simulink model "gg_plus_lc_platoon"  (R2019a)
settings: Solver=ode23t  StartTime=0.0  StopTime=70  FixedStep=0.1  MaxStep=0.01  RelTol=1e-3
InitFcn:
  | load vehStatesBus
libraries: simulink x120, powerlib_meascontrol x14, dspsigops x7, autolibshared x7
(part 1 of 7)
settings Model: Creator=fvall  LastModifiedBy=fvall
settings DebuggingCC: ReadBeforeWriteMsg=DisableAll  WriteAfterWriteMsg=DisableAll  WriteAfterReadMsg=DisableAll  MultiTaskDSMMsg=none
settings ModelReferenceCC: UpdateModelReferenceTargets=IfOutOfDate
settings SFSimCC: SFSimEcho=off

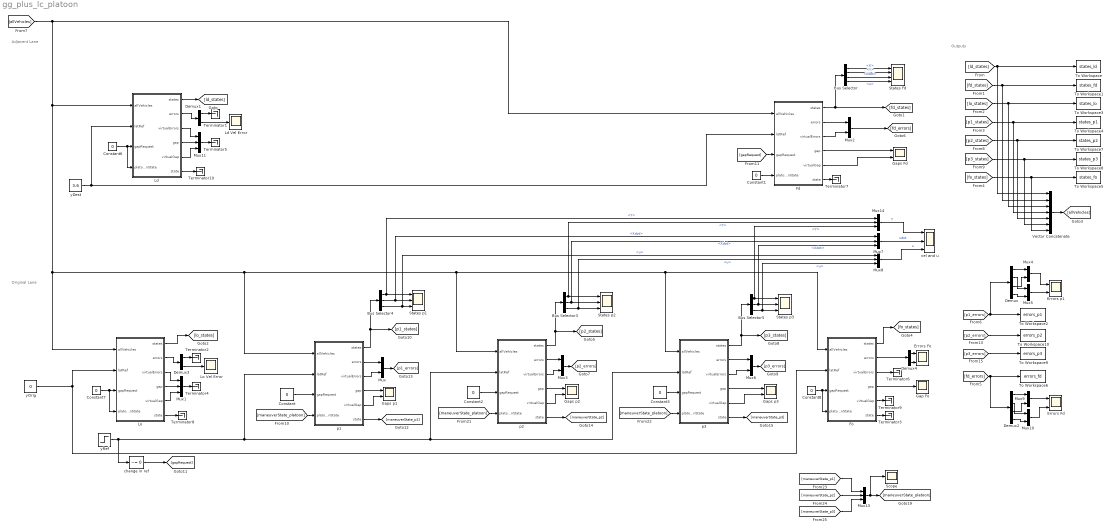
== system gg_plus_lc_platoon ==
  note: Adjacent Lane
  note: Outputs
  note: Original Lane
  Bus Selector : BusSelector  OutputSignals=X,Y,Xdot,u
  Bus Selector3 : BusSelector  OutputSignals=Y,Xdot,u
  Bus Selector4 : BusSelector  OutputSignals=Y,Xdot,u
  Bus Selector5 : BusSelector  OutputSignals=Y,Xdot,u
  Constant{,1..3,6..8} (7 alike) : Constant  Value=0
  Demux : Demux
  Demux1 : Demux  Outputs=2
  Demux2 : Demux
  Demux3 : Demux  Outputs=2
  Demux4 : Demux  Outputs=2
  Errors Fd : Scope  NumInputPorts=2
  Errors Fo : Scope  NumInputPorts=2
  Errors p1 : Scope  NumInputPorts=2
  Fd : Subsystem  mask{m=2000, lf=2.5, lr=2.5, maxAcceleration=4, minAcceleration=-8, maxJerk=40, minJerk=-50, maxDelta=0.43633, maxDeltaDot=0.16406, freeFlowVel=25, posInPlatoon=1, A=[0 1 25 0;0 -0.92 0 -25.1;0 0 0 1;0 -0.05 0 -2.875], B=[0;12;0;15], C=[1 0 0 0;0 0 0 1], x0=62.7512, vx0=25, y0=3.6, h=0.63, d0=0.5004, minHeadwayError=-100, maxHeadwayError=3, velFilterGain=10, Kd=1.5652, Kp=2.2775, Ki=0.75, velKi=0.5, velKp=1.5, hFilterGain=1, hFilterSaturation=0.5, vMin=16.25, maxComfAccel=2, minComfAccel=-2, maxComfJerk=10, minComfJerk=-10, strategy=2, hLc=1.9025, d0Lc=0.5004, Klat=[0.00909090909090922 0.00739381562390402 0.848484848484842 0.174418280834209], L=[12.1618468638973 6.0911647386398;-3.34743889176456 -72.8238882817198;1.29674659792577 4.97919690407453;0.0997536738638272 3.54315313610273]}
      mask prompts: m "autoblks_shared:autoblkVehBody3DofLat:blkPrm_m"; lf "autoblks_shared:autoblkVehBody3DofLat:blkPrm_a"; lr "autoblks_shared:autoblkVehBody3DofLat:blkPrm_b"; maxAcceleration "Max Acceleration"; minAcceleration "Min Acceleration"; maxJerk "Max Jerk"; minJerk "Min Jerk"; maxDelta "Max Delta"; maxDeltaDot "Max Delta Dot"; freeFlowVel "Free Flow Velocity"; posInPlatoon "Position in Platoon"; x0 "autoblks_shared:autoblkVehBody3DofLat:blkPrm_X_o"; vx0 "autoblks_shared:autoblkVehBody3DofLat:blkPrm_xdot_o"; y0 "autoblks_shared:autoblkVehBody3DofLat:blkPrm_Y_o"; h "Time Headway"; d0 "Standstill Gap"; minHeadwayError "Min Headway Error"; maxHeadwayError "Max Headway Error"; velFilterGain "Velocity Filter Gain"; hFilterGain "Headway Filter Gain"; hFilterSaturation "Headway Filter Saturation"; vMin "Min Velocity"; maxComfAccel "Max Comf Accel"; minComfAccel "Min Comf Accel"; maxComfJerk "Max Comf Jerk"; minComfJerk "Min Comf Jerk"; strategy "LC strategy"; hLc "Time Headway LC"; d0Lc "Standstill Gap LC"; Klat "Lat Controller Gain"; L "Observer Gain"
      mask TypeOptions m: Vehicle Body 3DOF Single Track/m
      mask TypeOptions lf: Vehicle Body 3DOF Single Track/a
      mask TypeOptions lr: Vehicle Body 3DOF Single Track/b
      mask TypeOptions maxDelta: Lateral Control/Saturation/UpperLimit
      mask TypeOptions maxDeltaDot: Lateral Control/Rate Limiter/RisingSlewLimit
      mask TypeOptions posInPlatoon: posInPlatoon/Value
      mask TypeOptions A:
      | Lateral Control/Full State
      | Observer/Gain3/Gain
      mask TypeOptions B:
      | Lateral Control/Full State
      | Observer/Gain/Gain
      mask TypeOptions C:
      | Lateral Control/Full State
      | Observer/Gain1/Gain
      mask TypeOptions x0: Vehicle Body 3DOF Single Track/X_o
      mask TypeOptions vx0: Vehicle Body 3DOF Single Track/xdot_o
      mask TypeOptions y0: Vehicle Body 3DOF Single Track/Y_o
      mask TypeOptions h:
      | Regular Vehicle
      | Following/Compute Errors/h/Value
      mask TypeOptions d0:
      | Regular Vehicle
      | Following/Compute Errors/d0/Value
      mask TypeOptions strategy: strategy/Value
      mask TypeOptions Klat: Lateral Control/Gain1/Gain
      mask TypeOptions L:
      | Lateral Control/Full State
      | Observer/Gain2/Gain
      mask DialogControl DescGroupVar Prompt: 3DOF Vehicle with ACC
      mask DialogControl DescTextVar Prompt: Vehicle with ACC. The vehicle model is Simulink's 3DOF single track vehicle body. The controller is a PID with constant headway including headway error saturation and filtered leader velocity.
      mask DialogControl VehParams Prompt: Vehicle Parameters
      mask DialogControl m Prompt: Vehicle mass, m [kg]:
      mask DialogControl lf Prompt: Longitudinal distance from center of mass to front axle, a [m]:
      mask DialogControl lr Prompt: Longitudinal distance from center of mass to rear axle, b [m]:
      mask DialogControl latLinearModel Prompt: Lat Linear Model
      mask DialogControl InitStates Prompt: Initial State
      mask DialogControl x0 Prompt: Initial inertial frame longitudinal position, X_o [m]:
      mask DialogControl vx0 Prompt: Initial longitudinal velocity, xdot_o [m/s]:
      mask DialogControl y0 Prompt: Initial inertial frame lateral displacement, Y_o [m]:
      mask DialogControl Container3 Prompt: Veh Following Parameters
      mask DialogControl VirtualFollParams Prompt: Virtual Veh Following Parameters
      mask DialogControl LCParams Prompt: Lane Change Params
  Fo : Subsystem  mask{m=2000, lf=2.5, lr=2.5, maxAcceleration=4, minAcceleration=-8, maxJerk=40, minJerk=-50, maxDelta=0.43633, maxDeltaDot=0.16406, freeFlowVel=25, posInPlatoon=1, A=[0 1 25 0;0 -0.92 0 -25.1;0 0 0 1;0 -0.05 0 -2.875], B=[0;12;0;15], C=[1 0 0 0;0 0 0 1], x0=0, vx0=25, y0=0, h=0.63, d0=0.5004, minHeadwayError=-100, maxHeadwayError=3, velFilterGain=10, Kd=1.5652, Kp=2.2775, Ki=0.75, velKi=0.5, velKp=1.5, hFilterGain=1, hFilterSaturation=0.5, vMin=16.25, maxComfAccel=2, minComfAccel=-2, maxComfJerk=10, minComfJerk=-10, strategy=2, hLc=1.9025, d0Lc=0.5004, Klat=[0.00909090909090922 0.00739381562390402 0.848484848484842 0.174418280834209], L=[12.1618468638973 6.0911647386398;-3.34743889176456 -72.8238882817198;1.29674659792577 4.97919690407453;0.0997536738638272 3.54315313610273]}
      mask prompts: m "autoblks_shared:autoblkVehBody3DofLat:blkPrm_m"; lf "autoblks_shared:autoblkVehBody3DofLat:blkPrm_a"; lr "autoblks_shared:autoblkVehBody3DofLat:blkPrm_b"; maxAcceleration "Max Acceleration"; minAcceleration "Min Acceleration"; maxJerk "Max Jerk"; minJerk "Min Jerk"; maxDelta "Max Delta"; maxDeltaDot "Max Delta Dot"; freeFlowVel "Free Flow Velocity"; posInPlatoon "Position in Platoon"; x0 "autoblks_shared:autoblkVehBody3DofLat:blkPrm_X_o"; vx0 "autoblks_shared:autoblkVehBody3DofLat:blkPrm_xdot_o"; y0 "autoblks_shared:autoblkVehBody3DofLat:blkPrm_Y_o"; h "Time Headway"; d0 "Standstill Gap"; minHeadwayError "Min Headway Error"; maxHeadwayError "Max Headway Error"; velFilterGain "Velocity Filter Gain"; hFilterGain "Headway Filter Gain"; hFilterSaturation "Headway Filter Saturation"; vMin "Min Velocity"; maxComfAccel "Max Comf Accel"; minComfAccel "Min Comf Accel"; maxComfJerk "Max Comf Jerk"; minComfJerk "Min Comf Jerk"; strategy "LC strategy"; hLc "Time Headway LC"; d0Lc "Standstill Gap LC"; Klat "Lat Controller Gain"; L "Observer Gain"
      mask TypeOptions m: Vehicle Body 3DOF Single Track/m
      mask TypeOptions lf: Vehicle Body 3DOF Single Track/a
      mask TypeOptions lr: Vehicle Body 3DOF Single Track/b
      mask TypeOptions maxDelta: Lateral Control/Saturation/UpperLimit
      mask TypeOptions maxDeltaDot: Lateral Control/Rate Limiter/RisingSlewLimit
      mask TypeOptions posInPlatoon: posInPlatoon/Value
      mask TypeOptions A:
      | Lateral Control/Full State
      | Observer/Gain3/Gain
      mask TypeOptions B:
      | Lateral Control/Full State
      | Observer/Gain/Gain
      mask TypeOptions C:
      | Lateral Control/Full State
      | Observer/Gain1/Gain
      mask TypeOptions x0: Vehicle Body 3DOF Single Track/X_o
      mask TypeOptions vx0: Vehicle Body 3DOF Single Track/xdot_o
      mask TypeOptions y0: Vehicle Body 3DOF Single Track/Y_o
      mask TypeOptions h:
      | Regular Vehicle
      | Following/Compute Errors/h/Value
      mask TypeOptions d0:
      | Regular Vehicle
      | Following/Compute Errors/d0/Value
      mask TypeOptions strategy: strategy/Value
      mask TypeOptions Klat: Lateral Control/Gain1/Gain
      mask TypeOptions L:
      | Lateral Control/Full State
      | Observer/Gain2/Gain
      mask DialogControl DescGroupVar Prompt: 3DOF Vehicle with ACC
      mask DialogControl DescTextVar Prompt: Vehicle with ACC. The vehicle model is Simulink's 3DOF single track vehicle body. The controller is a PID with constant headway including headway error saturation and filtered leader velocity.
      mask DialogControl VehParams Prompt: Vehicle Parameters
      mask DialogControl m Prompt: Vehicle mass, m [kg]:
      mask DialogControl lf Prompt: Longitudinal distance from center of mass to front axle, a [m]:
      mask DialogControl lr Prompt: Longitudinal distance from center of mass to rear axle, b [m]:
      mask DialogControl latLinearModel Prompt: Lat Linear Model
      mask DialogControl InitStates Prompt: Initial State
      mask DialogControl x0 Prompt: Initial inertial frame longitudinal position, X_o [m]:
      mask DialogControl vx0 Prompt: Initial longitudinal velocity, xdot_o [m/s]:
      mask DialogControl y0 Prompt: Initial inertial frame lateral displacement, Y_o [m]:
      mask DialogControl Container3 Prompt: Veh Following Parameters
      mask DialogControl VirtualFollParams Prompt: Virtual Veh Following Parameters
      mask DialogControl LCParams Prompt: Lane Change Params
  Gap Fo : Scope
  Gaps Fd : Scope  NumInputPorts=2
  Gaps p1 : Scope  NumInputPorts=2
  Gaps p2 : Scope  NumInputPorts=2
  Gaps p3 : Scope  NumInputPorts=2
  Ld : Subsystem  mask{m=2000, lf=2.5, lr=2.5, maxAcceleration=4, minAcceleration=-8, maxJerk=40, minJerk=-50, maxDelta=0.43633, maxDeltaDot=0.16406, freeFlowVel=25, posInPlatoon=1, A=[0 1 25 0;0 -0.92 0 -25.1;0 0 0 1;0 -0.05 0 -2.875], B=[0;12;0;15], C=[1 0 0 0;0 0 0 1], x0=84.0016, vx0=25, y0=3.6, h=0.63, d0=0.5004, minHeadwayError=-100, maxHeadwayError=3, velFilterGain=10, Kd=1.5652, Kp=2.2775, Ki=0.75, velKi=0.5, velKp=1.5, hFilterGain=1, hFilterSaturation=0.5, vMin=16.25, maxComfAccel=2, minComfAccel=-2, maxComfJerk=10, minComfJerk=-10, strategy=2, hLc=1.9025, d0Lc=0.5004, Klat=[0.00909090909090922 0.00739381562390402 0.848484848484842 0.174418280834209], L=[12.1618468638973 6.0911647386398;-3.34743889176456 -72.8238882817198;1.29674659792577 4.97919690407453;0.0997536738638272 3.54315313610273]}
      mask prompts: m "autoblks_shared:autoblkVehBody3DofLat:blkPrm_m"; lf "autoblks_shared:autoblkVehBody3DofLat:blkPrm_a"; lr "autoblks_shared:autoblkVehBody3DofLat:blkPrm_b"; maxAcceleration "Max Acceleration"; minAcceleration "Min Acceleration"; maxJerk "Max Jerk"; minJerk "Min Jerk"; maxDelta "Max Delta"; maxDeltaDot "Max Delta Dot"; freeFlowVel "Free Flow Velocity"; posInPlatoon "Position in Platoon"; x0 "autoblks_shared:autoblkVehBody3DofLat:blkPrm_X_o"; vx0 "autoblks_shared:autoblkVehBody3DofLat:blkPrm_xdot_o"; y0 "autoblks_shared:autoblkVehBody3DofLat:blkPrm_Y_o"; h "Time Headway"; d0 "Standstill Gap"; minHeadwayError "Min Headway Error"; maxHeadwayError "Max Headway Error"; velFilterGain "Velocity Filter Gain"; hFilterGain "Headway Filter Gain"; hFilterSaturation "Headway Filter Saturation"; vMin "Min Velocity"; maxComfAccel "Max Comf Accel"; minComfAccel "Min Comf Accel"; maxComfJerk "Max Comf Jerk"; minComfJerk "Min Comf Jerk"; strategy "LC strategy"; hLc "Time Headway LC"; d0Lc "Standstill Gap LC"; Klat "Lat Controller Gain"; L "Observer Gain"
      mask TypeOptions m: Vehicle Body 3DOF Single Track/m
      mask TypeOptions lf: Vehicle Body 3DOF Single Track/a
      mask TypeOptions lr: Vehicle Body 3DOF Single Track/b
      mask TypeOptions maxDelta: Lateral Control/Saturation/UpperLimit
      mask TypeOptions maxDeltaDot: Lateral Control/Rate Limiter/RisingSlewLimit
      mask TypeOptions posInPlatoon: posInPlatoon/Value
      mask TypeOptions A:
      | Lateral Control/Full State
      | Observer/Gain3/Gain
      mask TypeOptions B:
      | Lateral Control/Full State
      | Observer/Gain/Gain
      mask TypeOptions C:
      | Lateral Control/Full State
      | Observer/Gain1/Gain
      mask TypeOptions x0: Vehicle Body 3DOF Single Track/X_o
      mask TypeOptions vx0: Vehicle Body 3DOF Single Track/xdot_o
      mask TypeOptions y0: Vehicle Body 3DOF Single Track/Y_o
      mask TypeOptions h:
      | Regular Vehicle
      | Following/Compute Errors/h/Value
      mask TypeOptions d0:
      | Regular Vehicle
      | Following/Compute Errors/d0/Value
      mask TypeOptions strategy: strategy/Value
      mask TypeOptions Klat: Lateral Control/Gain1/Gain
      mask TypeOptions L:
      | Lateral Control/Full State
      | Observer/Gain2/Gain
      mask DialogControl DescGroupVar Prompt: 3DOF Vehicle with ACC
      mask DialogControl DescTextVar Prompt: Vehicle with ACC. The vehicle model is Simulink's 3DOF single track vehicle body. The controller is a PID with constant headway including headway error saturation and filtered leader velocity.
      mask DialogControl VehParams Prompt: Vehicle Parameters
      mask DialogControl m Prompt: Vehicle mass, m [kg]:
      mask DialogControl lf Prompt: Longitudinal distance from center of mass to front axle, a [m]:
      mask DialogControl lr Prompt: Longitudinal distance from center of mass to rear axle, b [m]:
      mask DialogControl latLinearModel Prompt: Lat Linear Model
      mask DialogControl InitStates Prompt: Initial State
      mask DialogControl x0 Prompt: Initial inertial frame longitudinal position, X_o [m]:
      mask DialogControl vx0 Prompt: Initial longitudinal velocity, xdot_o [m/s]:
      mask DialogControl y0 Prompt: Initial inertial frame lateral displacement, Y_o [m]:
      mask DialogControl Container3 Prompt: Veh Following Parameters
      mask DialogControl VirtualFollParams Prompt: Virtual Veh Following Parameters
      mask DialogControl LCParams Prompt: Lane Change Params
  Ld Vel Error : Scope
  Lo : Subsystem  mask{m=2000, lf=2.5, lr=2.5, maxAcceleration=4, minAcceleration=-8, maxJerk=40, minJerk=-50, maxDelta=0.43633, maxDeltaDot=0.16406, freeFlowVel=25, posInPlatoon=1, A=[0 1 25 0;0 -0.92 0 -25.1;0 0 0 1;0 -0.05 0 -2.875], B=[0;12;0;15], C=[1 0 0 0;0 0 0 1], x0=85.0016, vx0=25, y0=0, h=0.63, d0=0.5004, minHeadwayError=-100, maxHeadwayError=3, velFilterGain=10, Kd=1.5652, Kp=2.2775, Ki=0.75, velKi=0.5, velKp=1.5, hFilterGain=1, hFilterSaturation=0.5, vMin=16.25, maxComfAccel=2, minComfAccel=-2, maxComfJerk=10, minComfJerk=-10, strategy=2, hLc=1.9025, d0Lc=0.5004, Klat=[0.00909090909090922 0.00739381562390402 0.848484848484842 0.174418280834209], L=[12.1618468638973 6.0911647386398;-3.34743889176456 -72.8238882817198;1.29674659792577 4.97919690407453;0.0997536738638272 3.54315313610273]}
      mask prompts: m "autoblks_shared:autoblkVehBody3DofLat:blkPrm_m"; lf "autoblks_shared:autoblkVehBody3DofLat:blkPrm_a"; lr "autoblks_shared:autoblkVehBody3DofLat:blkPrm_b"; maxAcceleration "Max Acceleration"; minAcceleration "Min Acceleration"; maxJerk "Max Jerk"; minJerk "Min Jerk"; maxDelta "Max Delta"; maxDeltaDot "Max Delta Dot"; freeFlowVel "Free Flow Velocity"; posInPlatoon "Position in Platoon"; x0 "autoblks_shared:autoblkVehBody3DofLat:blkPrm_X_o"; vx0 "autoblks_shared:autoblkVehBody3DofLat:blkPrm_xdot_o"; y0 "autoblks_shared:autoblkVehBody3DofLat:blkPrm_Y_o"; h "Time Headway"; d0 "Standstill Gap"; minHeadwayError "Min Headway Error"; maxHeadwayError "Max Headway Error"; velFilterGain "Velocity Filter Gain"; hFilterGain "Headway Filter Gain"; hFilterSaturation "Headway Filter Saturation"; vMin "Min Velocity"; maxComfAccel "Max Comf Accel"; minComfAccel "Min Comf Accel"; maxComfJerk "Max Comf Jerk"; minComfJerk "Min Comf Jerk"; strategy "LC strategy"; hLc "Time Headway LC"; d0Lc "Standstill Gap LC"; Klat "Lat Controller Gain"; L "Observer Gain"
      mask TypeOptions m: Vehicle Body 3DOF Single Track/m
      mask TypeOptions lf: Vehicle Body 3DOF Single Track/a
      mask TypeOptions lr: Vehicle Body 3DOF Single Track/b
      mask TypeOptions maxDelta: Lateral Control/Saturation/UpperLimit
      mask TypeOptions maxDeltaDot: Lateral Control/Rate Limiter/RisingSlewLimit
      mask TypeOptions posInPlatoon: posInPlatoon/Value
      mask TypeOptions A:
      | Lateral Control/Full State
      | Observer/Gain3/Gain
      mask TypeOptions B:
      | Lateral Control/Full State
      | Observer/Gain/Gain
      mask TypeOptions C:
      | Lateral Control/Full State
      | Observer/Gain1/Gain
      mask TypeOptions x0: Vehicle Body 3DOF Single Track/X_o
      mask TypeOptions vx0: Vehicle Body 3DOF Single Track/xdot_o
      mask TypeOptions y0: Vehicle Body 3DOF Single Track/Y_o
      mask TypeOptions h:
      | Regular Vehicle
      | Following/Compute Errors/h/Value
      mask TypeOptions d0:
      | Regular Vehicle
      | Following/Compute Errors/d0/Value
      mask TypeOptions strategy: strategy/Value
      mask TypeOptions Klat: Lateral Control/Gain1/Gain
      mask TypeOptions L:
      | Lateral Control/Full State
      | Observer/Gain2/Gain
      mask DialogControl DescGroupVar Prompt: 3DOF Vehicle with ACC
      mask DialogControl DescTextVar Prompt: Vehicle with ACC. The vehicle model is Simulink's 3DOF single track vehicle body. The controller is a PID with constant headway including headway error saturation and filtered leader velocity.
      mask DialogControl VehParams Prompt: Vehicle Parameters
      mask DialogControl m Prompt: Vehicle mass, m [kg]:
      mask DialogControl lf Prompt: Longitudinal distance from center of mass to front axle, a [m]:
      mask DialogControl lr Prompt: Longitudinal distance from center of mass to rear axle, b [m]:
      mask DialogControl latLinearModel Prompt: Lat Linear Model
      mask DialogControl InitStates Prompt: Initial State
      mask DialogControl x0 Prompt: Initial inertial frame longitudinal position, X_o [m]:
      mask DialogControl vx0 Prompt: Initial longitudinal velocity, xdot_o [m/s]:
      mask DialogControl y0 Prompt: Initial inertial frame lateral displacement, Y_o [m]:
      mask DialogControl Container3 Prompt: Veh Following Parameters
      mask DialogControl VirtualFollParams Prompt: Virtual Veh Following Parameters
      mask DialogControl LCParams Prompt: Lane Change Params
  Lo Vel Error : Scope
  Mux{,2..6,9..10} (8 alike) : Mux  Inputs=2
  Mux{1,7..8,11,13..14} (6 alike) : Mux  Inputs=3
  Scope : Scope
  States Fd : Scope  NumInputPorts=4
  States p1 : Scope  NumInputPorts=3
  States p2 : Scope  NumInputPorts=3
  States p3 : Scope  NumInputPorts=3
  Terminator{1..10} (10 alike) : Terminator
  To Workspace : ToWorkspace  VariableName=states_ld  SaveFormat=Timeseries  SampleTime=-1
  To Workspace1 : ToWorkspace  VariableName=states_fd  SaveFormat=Timeseries  SampleTime=-1
  To Workspace10 : ToWorkspace  VariableName=errors_p2  SampleTime=-1
  To Workspace2 : ToWorkspace  VariableName=errors_p1  SampleTime=-1
  To Workspace3 : ToWorkspace  VariableName=states_lo  SaveFormat=Timeseries  SampleTime=-1
  To Workspace4 : ToWorkspace  VariableName=states_p1  SaveFormat=Timeseries  SampleTime=-1
  To Workspace5 : ToWorkspace  VariableName=states_fo  SaveFormat=Timeseries  SampleTime=-1
  To Workspace6 : ToWorkspace  VariableName=errors_fd  SampleTime=-1
  To Workspace7 : ToWorkspace  VariableName=states_p2  SaveFormat=Timeseries  SampleTime=-1
  To Workspace8 : ToWorkspace  VariableName=states_p3  SaveFormat=Timeseries  SampleTime=-1
  To Workspace9 : ToWorkspace  VariableName=errors_p3  SampleTime=-1
  Vector Concatenate : Concatenate  NumInputs=7
  change in ref : simulink/Logic and Bit Operations/Compare To Constant  relop=~=  const=0  OutDataTypeStr=boolean
  p1 : Subsystem  mask{m=2000, lf=2.5, lr=2.5, maxAcceleration=4, minAcceleration=-8, maxJerk=40, minJerk=-50, maxDelta=0.43633, maxDeltaDot=0.16406, freeFlowVel=25, posInPlatoon=1, A=[0 1 25 0;0 -0.92 0 -25.1;0 0 0 1;0 -0.05 0 -2.875], B=[0;12;0;15], C=[1 0 0 0;0 0 0 1], x0=63.7512, vx0=25, y0=0, h=0.63, d0=0.5004, minHeadwayError=-100, maxHeadwayError=3, velFilterGain=10, Kd=1.5652, Kp=2.2775, Ki=0.75, velKi=0.5, velKp=1.5, hFilterGain=1, hFilterSaturation=0.5, vMin=16.25, maxComfAccel=2, minComfAccel=-2, maxComfJerk=10, minComfJerk=-10, strategy=2, hLc=1.9025, d0Lc=0.5004, Klat=[0.00909090909090922 0.00739381562390402 0.848484848484842 0.174418280834209], L=[12.1618468638973 6.0911647386398;-3.34743889176456 -72.8238882817198;1.29674659792577 4.97919690407453;0.0997536738638272 3.54315313610273]}
      mask prompts: m "autoblks_shared:autoblkVehBody3DofLat:blkPrm_m"; lf "autoblks_shared:autoblkVehBody3DofLat:blkPrm_a"; lr "autoblks_shared:autoblkVehBody3DofLat:blkPrm_b"; maxAcceleration "Max Acceleration"; minAcceleration "Min Acceleration"; maxJerk "Max Jerk"; minJerk "Min Jerk"; maxDelta "Max Delta"; maxDeltaDot "Max Delta Dot"; freeFlowVel "Free Flow Velocity"; posInPlatoon "Position in Platoon"; x0 "autoblks_shared:autoblkVehBody3DofLat:blkPrm_X_o"; vx0 "autoblks_shared:autoblkVehBody3DofLat:blkPrm_xdot_o"; y0 "autoblks_shared:autoblkVehBody3DofLat:blkPrm_Y_o"; h "Time Headway"; d0 "Standstill Gap"; minHeadwayError "Min Headway Error"; maxHeadwayError "Max Headway Error"; velFilterGain "Velocity Filter Gain"; hFilterGain "Headway Filter Gain"; hFilterSaturation "Headway Filter Saturation"; vMin "Min Velocity"; maxComfAccel "Max Comf Accel"; minComfAccel "Min Comf Accel"; maxComfJerk "Max Comf Jerk"; minComfJerk "Min Comf Jerk"; strategy "LC strategy"; hLc "Time Headway LC"; d0Lc "Standstill Gap LC"; Klat "Lat Controller Gain"; L "Observer Gain"
      mask TypeOptions m: Vehicle Body 3DOF Single Track/m
      mask TypeOptions lf: Vehicle Body 3DOF Single Track/a
      mask TypeOptions lr: Vehicle Body 3DOF Single Track/b
      mask TypeOptions maxDelta: Lateral Control/Saturation/UpperLimit
      mask TypeOptions maxDeltaDot: Lateral Control/Rate Limiter/RisingSlewLimit
      mask TypeOptions posInPlatoon: posInPlatoon/Value
      mask TypeOptions A:
      | Lateral Control/Full State
      | Observer/Gain3/Gain
      mask TypeOptions B:
      | Lateral Control/Full State
      | Observer/Gain/Gain
      mask TypeOptions C:
      | Lateral Control/Full State
      | Observer/Gain1/Gain
      mask TypeOptions x0: Vehicle Body 3DOF Single Track/X_o
      mask TypeOptions vx0: Vehicle Body 3DOF Single Track/xdot_o
      mask TypeOptions y0: Vehicle Body 3DOF Single Track/Y_o
      mask TypeOptions h:
      | Regular Vehicle
      | Following/Compute Errors/h/Value
      mask TypeOptions d0:
      | Regular Vehicle
      | Following/Compute Errors/d0/Value
      mask TypeOptions strategy: strategy/Value
      mask TypeOptions Klat: Lateral Control/Gain1/Gain
      mask TypeOptions L:
      | Lateral Control/Full State
      | Observer/Gain2/Gain
      mask DialogControl DescGroupVar Prompt: 3DOF Vehicle with ACC
      mask DialogControl DescTextVar Prompt: Vehicle with ACC. The vehicle model is Simulink's 3DOF single track vehicle body. The controller is a PID with constant headway including headway error saturation and filtered leader velocity.
      mask DialogControl VehParams Prompt: Vehicle Parameters
      mask DialogControl m Prompt: Vehicle mass, m [kg]:
      mask DialogControl lf Prompt: Longitudinal distance from center of mass to front axle, a [m]:
      mask DialogControl lr Prompt: Longitudinal distance from center of mass to rear axle, b [m]:
      mask DialogControl latLinearModel Prompt: Lat Linear Model
      mask DialogControl InitStates Prompt: Initial State
      mask DialogControl x0 Prompt: Initial inertial frame longitudinal position, X_o [m]:
      mask DialogControl vx0 Prompt: Initial longitudinal velocity, xdot_o [m/s]:
      mask DialogControl y0 Prompt: Initial inertial frame lateral displacement, Y_o [m]:
      mask DialogControl Container3 Prompt: Veh Following Parameters
      mask DialogControl VirtualFollParams Prompt: Virtual Veh Following Parameters
      mask DialogControl LCParams Prompt: Lane Change Params
  p2 : Subsystem  mask{m=2000, lf=2.5, lr=2.5, maxAcceleration=4, minAcceleration=-8, maxJerk=40, minJerk=-50, maxDelta=0.43633, maxDeltaDot=0.16406, freeFlowVel=25, posInPlatoon=2, A=[0 1 25 0;0 -0.92 0 -25.1;0 0 0 1;0 -0.05 0 -2.875], B=[0;12;0;15], C=[1 0 0 0;0 0 0 1], x0=42.5008, vx0=25, y0=0, h=0.63, d0=0.5004, minHeadwayError=-100, maxHeadwayError=3, velFilterGain=10, Kd=1.5652, Kp=2.2775, Ki=0.75, velKi=0.5, velKp=1.5, hFilterGain=1, hFilterSaturation=0.5, vMin=16.25, maxComfAccel=2, minComfAccel=-2, maxComfJerk=10, minComfJerk=-10, strategy=2, hLc=1.9025, d0Lc=0.5004, Klat=[0.00909090909090922 0.00739381562390402 0.848484848484842 0.174418280834209], L=[12.1618468638973 6.0911647386398;-3.34743889176456 -72.8238882817198;1.29674659792577 4.97919690407453;0.0997536738638272 3.54315313610273]}
      mask prompts: m "autoblks_shared:autoblkVehBody3DofLat:blkPrm_m"; lf "autoblks_shared:autoblkVehBody3DofLat:blkPrm_a"; lr "autoblks_shared:autoblkVehBody3DofLat:blkPrm_b"; maxAcceleration "Max Acceleration"; minAcceleration "Min Acceleration"; maxJerk "Max Jerk"; minJerk "Min Jerk"; maxDelta "Max Delta"; maxDeltaDot "Max Delta Dot"; freeFlowVel "Free Flow Velocity"; posInPlatoon "Position in Platoon"; x0 "autoblks_shared:autoblkVehBody3DofLat:blkPrm_X_o"; vx0 "autoblks_shared:autoblkVehBody3DofLat:blkPrm_xdot_o"; y0 "autoblks_shared:autoblkVehBody3DofLat:blkPrm_Y_o"; h "Time Headway"; d0 "Standstill Gap"; minHeadwayError "Min Headway Error"; maxHeadwayError "Max Headway Error"; velFilterGain "Velocity Filter Gain"; hFilterGain "Headway Filter Gain"; hFilterSaturation "Headway Filter Saturation"; vMin "Min Velocity"; maxComfAccel "Max Comf Accel"; minComfAccel "Min Comf Accel"; maxComfJerk "Max Comf Jerk"; minComfJerk "Min Comf Jerk"; strategy "LC strategy"; hLc "Time Headway LC"; d0Lc "Standstill Gap LC"; Klat "Lat Controller Gain"; L "Observer Gain"
      mask TypeOptions m: Vehicle Body 3DOF Single Track/m
      mask TypeOptions lf: Vehicle Body 3DOF Single Track/a
      mask TypeOptions lr: Vehicle Body 3DOF Single Track/b
      mask TypeOptions maxDelta: Lateral Control/Saturation/UpperLimit
      mask TypeOptions maxDeltaDot: Lateral Control/Rate Limiter/RisingSlewLimit
      mask TypeOptions posInPlatoon: posInPlatoon/Value
      mask TypeOptions A:
      | Lateral Control/Full State
      | Observer/Gain3/Gain
      mask TypeOptions B:
      | Lateral Control/Full State
      | Observer/Gain/Gain
      mask TypeOptions C:
      | Lateral Control/Full State
      | Observer/Gain1/Gain
      mask TypeOptions x0: Vehicle Body 3DOF Single Track/X_o
      mask TypeOptions vx0: Vehicle Body 3DOF Single Track/xdot_o
      mask TypeOptions y0: Vehicle Body 3DOF Single Track/Y_o
      mask TypeOptions h:
      | Regular Vehicle
      | Following/Compute Errors/h/Value
      mask TypeOptions d0:
      | Regular Vehicle
      | Following/Compute Errors/d0/Value
      mask TypeOptions strategy: strategy/Value
      mask TypeOptions Klat: Lateral Control/Gain1/Gain
      mask TypeOptions L:
      | Lateral Control/Full State
      | Observer/Gain2/Gain
      mask DialogControl DescGroupVar Prompt: 3DOF Vehicle with ACC
      mask DialogControl DescTextVar Prompt: Vehicle with ACC. The vehicle model is Simulink's 3DOF single track vehicle body. The controller is a PID with constant headway including headway error saturation and filtered leader velocity.
      mask DialogControl VehParams Prompt: Vehicle Parameters
      mask DialogControl m Prompt: Vehicle mass, m [kg]:
      mask DialogControl lf Prompt: Longitudinal distance from center of mass to front axle, a [m]:
      mask DialogControl lr Prompt: Longitudinal distance from center of mass to rear axle, b [m]:
      mask DialogControl latLinearModel Prompt: Lat Linear Model
      mask DialogControl InitStates Prompt: Initial State
      mask DialogControl x0 Prompt: Initial inertial frame longitudinal position, X_o [m]:
      mask DialogControl vx0 Prompt: Initial longitudinal velocity, xdot_o [m/s]:
      mask DialogControl y0 Prompt: Initial inertial frame lateral displacement, Y_o [m]:
      mask DialogControl Container3 Prompt: Veh Following Parameters
      mask DialogControl VirtualFollParams Prompt: Virtual Veh Following Parameters
      mask DialogControl LCParams Prompt: Lane Change Params
  p3 : Subsystem  mask{m=2000, lf=2.5, lr=2.5, maxAcceleration=4, minAcceleration=-8, maxJerk=40, minJerk=-50, maxDelta=0.43633, maxDeltaDot=0.16406, freeFlowVel=25, posInPlatoon=3, A=[0 1 25 0;0 -0.92 0 -25.1;0 0 0 1;0 -0.05 0 -2.875], B=[0;12;0;15], C=[1 0 0 0;0 0 0 1], x0=21.2504, vx0=25, y0=0, h=0.63, d0=0.5004, minHeadwayError=-100, maxHeadwayError=3, velFilterGain=10, Kd=1.5652, Kp=2.2775, Ki=0.75, velKi=0.5, velKp=1.5, hFilterGain=1, hFilterSaturation=0.5, vMin=16.25, maxComfAccel=2, minComfAccel=-2, maxComfJerk=10, minComfJerk=-10, strategy=2, hLc=1.9025, d0Lc=0.5004, Klat=[0.00909090909090922 0.00739381562390402 0.848484848484842 0.174418280834209], L=[12.1618468638973 6.0911647386398;-3.34743889176456 -72.8238882817198;1.29674659792577 4.97919690407453;0.0997536738638272 3.54315313610273]}
      mask prompts: m "autoblks_shared:autoblkVehBody3DofLat:blkPrm_m"; lf "autoblks_shared:autoblkVehBody3DofLat:blkPrm_a"; lr "autoblks_shared:autoblkVehBody3DofLat:blkPrm_b"; maxAcceleration "Max Acceleration"; minAcceleration "Min Acceleration"; maxJerk "Max Jerk"; minJerk "Min Jerk"; maxDelta "Max Delta"; maxDeltaDot "Max Delta Dot"; freeFlowVel "Free Flow Velocity"; posInPlatoon "Position in Platoon"; x0 "autoblks_shared:autoblkVehBody3DofLat:blkPrm_X_o"; vx0 "autoblks_shared:autoblkVehBody3DofLat:blkPrm_xdot_o"; y0 "autoblks_shared:autoblkVehBody3DofLat:blkPrm_Y_o"; h "Time Headway"; d0 "Standstill Gap"; minHeadwayError "Min Headway Error"; maxHeadwayError "Max Headway Error"; velFilterGain "Velocity Filter Gain"; hFilterGain "Headway Filter Gain"; hFilterSaturation "Headway Filter Saturation"; vMin "Min Velocity"; maxComfAccel "Max Comf Accel"; minComfAccel "Min Comf Accel"; maxComfJerk "Max Comf Jerk"; minComfJerk "Min Comf Jerk"; strategy "LC strategy"; hLc "Time Headway LC"; d0Lc "Standstill Gap LC"; Klat "Lat Controller Gain"; L "Observer Gain"
      mask TypeOptions m: Vehicle Body 3DOF Single Track/m
      mask TypeOptions lf: Vehicle Body 3DOF Single Track/a
      mask TypeOptions lr: Vehicle Body 3DOF Single Track/b
      mask TypeOptions maxDelta: Lateral Control/Saturation/UpperLimit
      mask TypeOptions maxDeltaDot: Lateral Control/Rate Limiter/RisingSlewLimit
      mask TypeOptions posInPlatoon: posInPlatoon/Value
      mask TypeOptions A:
      | Lateral Control/Full State
      | Observer/Gain3/Gain
      mask TypeOptions B:
      | Lateral Control/Full State
      | Observer/Gain/Gain
      mask TypeOptions C:
      | Lateral Control/Full State
      | Observer/Gain1/Gain
      mask TypeOptions x0: Vehicle Body 3DOF Single Track/X_o
      mask TypeOptions vx0: Vehicle Body 3DOF Single Track/xdot_o
      mask TypeOptions y0: Vehicle Body 3DOF Single Track/Y_o
      mask TypeOptions h:
      | Regular Vehicle
      | Following/Compute Errors/h/Value
      mask TypeOptions d0:
      | Regular Vehicle
      | Following/Compute Errors/d0/Value
      mask TypeOptions strategy: strategy/Value
      mask TypeOptions Klat: Lateral Control/Gain1/Gain
      mask TypeOptions L:
      | Lateral Control/Full State
      | Observer/Gain2/Gain
      mask DialogControl DescGroupVar Prompt: 3DOF Vehicle with ACC
      mask DialogControl DescTextVar Prompt: Vehicle with ACC. The vehicle model is Simulink's 3DOF single track vehicle body. The controller is a PID with constant headway including headway error saturation and filtered leader velocity.
      mask DialogControl VehParams Prompt: Vehicle Parameters
      mask DialogControl m Prompt: Vehicle mass, m [kg]:
      mask DialogControl lf Prompt: Longitudinal distance from center of mass to front axle, a [m]:
      mask DialogControl lr Prompt: Longitudinal distance from center of mass to rear axle, b [m]:
      mask DialogControl latLinearModel Prompt: Lat Linear Model
      mask DialogControl InitStates Prompt: Initial State
      mask DialogControl x0 Prompt: Initial inertial frame longitudinal position, X_o [m]:
      mask DialogControl vx0 Prompt: Initial longitudinal velocity, xdot_o [m/s]:
      mask DialogControl y0 Prompt: Initial inertial frame lateral displacement, Y_o [m]:
      mask DialogControl Container3 Prompt: Veh Following Parameters
      mask DialogControl VirtualFollParams Prompt: Virtual Veh Following Parameters
      mask DialogControl LCParams Prompt: Lane Change Params
  vel and u : Scope  NumInputPorts=3
  yDest : Constant  Value=3.6
  yOrig : Constant  Value=0
  yRef : Step  Time=5  After=3.6  SampleTime=0
  wires:
  Lo/2(errors) -> Demux3/1
  Fo/3(virtualErrors) -> Terminator6/1
  Lo/5(virtualGap) -> Mux1/3
  [p1_errors] -> To Workspace2/1, Demux/1
  Lo/6(state) -> Terminator8/1
  Demux3/1 -> Terminator2/1
  Mux5/1 -> Errors p1/2
  Demux4/2 -> Errors Fo/2
  p1/3(virtualErrors) -> Mux/2
  Demux3/2 -> Lo Vel Error/1
  Bus Selector4/3 -> States p1/3, Mux8/1  "<u>"
  p1/5(virtualGap) -> Gaps p1/2
  Mux1/1 -> Terminator4/1
  Demux2/2 -> Mux10/1
  Lo/3(virtualErrors) -> Mux1/1
  Mux/1 -> [p1_errors]
  Demux/3 -> Mux4/2
  Fo/5(virtualGap) -> Terminator9/1
  Demux/1 -> Mux4/1
  [fo_states] -> To Workspace5/1, Vector Concatenate/7
  Demux2/1 -> Mux9/1
  Demux/4 -> Mux5/2
  [ld_states] -> To Workspace/1, Vector Concatenate/1
  [p1_states] -> Vector Concatenate/4, To Workspace4/1
  [fd_errors] -> Demux2/1, To Workspace6/1
  Demux2/4 -> Mux10/2
  change in ref/1 -> [gapRequest]
  Demux2/3 -> Mux9/2
  Fd/3(virtualErrors) -> Mux2/2
  Demux/2 -> Mux5/1
  Mux9/1 -> Errors Fd/1
  Demux4/1 -> Errors Fo/1
  Mux10/1 -> Errors Fd/2
  p1/1(states) -> Bus Selector4/1, [p1_states]
  Constant7/1 -> Lo/4(platoonState), Lo/3(gapRequest)
  Fd/2(errors) -> Mux2/1
  Fo/4(gap) -> Gap Fo/1
  Constant8/1 -> Fo/3(gapRequest), Fo/4(platoonState)
  Fo/1(states) -> [fo_states]
  [lo_states] -> To Workspace3/1, Vector Concatenate/3
  Fo/2(errors) -> Demux4/1
  Constant6/1 -> Ld/3(gapRequest), Ld/4(platoonState)
  Mux2/1 -> [fd_errors]
  Bus Selector/3 -> States Fd/3  "<Xdot>"
  Lo/1(states) -> [lo_states]
  p1/4(gap) -> Gaps p1/1
  [fd_states] -> To Workspace1/1, Vector Concatenate/2
  Mux4/1 -> Errors p1/1
  Bus Selector/4 -> States Fd/4  "<u>"
  Fd/5(virtualGap) -> Gaps Fd/2
  Bus Selector/1 -> States Fd/1  "<X>"
  Fd/4(gap) -> Gaps Fd/1
  Fd/1(states) -> Bus Selector/1, [fd_states]
  Fd/6(state) -> Terminator7/1
  p1/2(errors) -> Mux/1
  Ld/1(states) -> [ld_states]
  Bus Selector4/2 -> States p1/2, Mux7/1  "<Xdot>"
  yRef/1 -> change in ref/1, p1/2(latRef), p2/2(latRef), p3/2(latRef)
  yDest/1 -> Ld/2(latRef), Fd/2(latRef)
  yOrig/1 -> Fo/2(latRef), Lo/2(latRef)
  Bus Selector/2 -> States Fd/2  "<Y>"
  [allVehicles] -> Fd/1(allVehicles), Ld/1(allVehicles), Lo/1(allVehicles), p1/1(allVehicles), p2/1(allVehicles), p3/1(allVehicles), Fo/1(allVehicles)
  Vector Concatenate/1 -> [allVehicles]
  p2/4(gap) -> Gaps p2/1
  p2/3(virtualErrors) -> Mux3/2
  Bus Selector3/3 -> Mux8/2, States p2/3  "<u>"
  p2/5(virtualGap) -> Gaps p2/2
  p2/1(states) -> Bus Selector3/1, [p2_states]
  p2/2(errors) -> Mux3/1
  Mux3/1 -> [p2_errors]
  Bus Selector3/2 -> Mux7/2, States p2/2  "<Xdot>"
  Bus Selector3/1 -> Mux14/2, States p2/1  "<Y>"
  Bus Selector5/2 -> Mux7/3, States p3/2  "<Xdot>"
  Mux6/1 -> [p3_errors]
  Bus Selector5/1 -> Mux14/3, States p3/1  "<Y>"
  p3/2(errors) -> Mux6/1
  p3/3(virtualErrors) -> Mux6/2
  p3/1(states) -> Bus Selector5/1, [p3_states]
  p3/5(virtualGap) -> Gaps p3/2
  p3/4(gap) -> Gaps p3/1
  Bus Selector5/3 -> Mux8/3, States p3/3  "<u>"
  [p2_states] -> Vector Concatenate/5, To Workspace7/1
  [p3_states] -> Vector Concatenate/6, To Workspace8/1
  [p3_errors] -> To Workspace9/1
  [p2_errors] -> To Workspace10/1
  Mux7/1 -> vel and u/2  "xdot"
  Mux8/1 -> vel and u/3  "u"
  [gapRequest] -> Fd/3(gapRequest)
  p1/6(state) -> [maneuverState_p1]
  p2/6(state) -> [maneuverState_p2]
  p3/6(state) -> [maneuverState_p3]
  Constant/1 -> p1/3(gapRequest)
  Constant2/1 -> p2/3(gapRequest)
  Constant3/1 -> p3/3(gapRequest)
  [maneuverState_platoon] -> p1/4(platoonState)
  [maneuverState_platoon] -> p2/4(platoonState)
  [maneuverState_platoon] -> p3/4(platoonState)
  Fo/6(state) -> Terminator3/1
  Constant1/1 -> Fd/4(platoonState)
  Lo/4(gap) -> Mux1/2
  Demux1/2 -> Ld Vel Error/1
  Ld/2(errors) -> Demux1/1
  Demux1/1 -> Terminator1/1
  Ld/4(gap) -> Mux11/2
  Mux11/1 -> Terminator5/1
  Ld/6(state) -> Terminator10/1
  Ld/5(virtualGap) -> Mux11/3
  Ld/3(virtualErrors) -> Mux11/1
  [maneuverState_p2] -> Mux13/2
  [maneuverState_p1] -> Mux13/1
  [maneuverState_p3] -> Mux13/3
  Mux13/1 -> Scope/1, [maneuverState_platoon]
  Bus Selector4/1 -> Mux14/1, States p1/1  "<Y>"
  Mux14/1 -> vel and u/1  "Y"

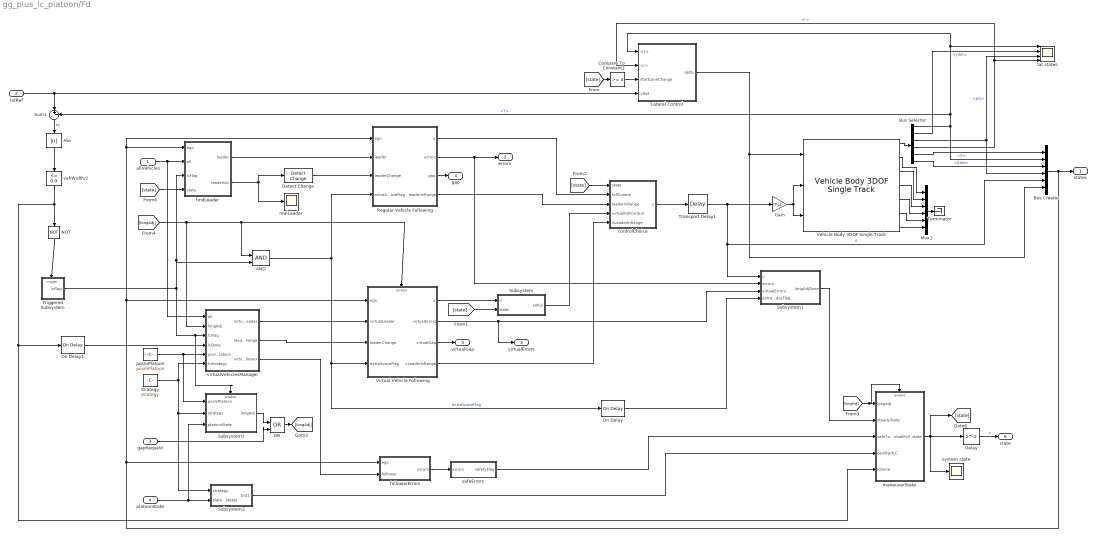
== system gg_plus_lc_platoon/Fd ==
  allVehicles : Inport
  latRef : Inport  Port=2
  gapRequest : Inport  Port=3
  platoonState : Inport  Port=4
  AND : Logic  IconShape=distinctive  AllPortsSameDT=off  OutDataTypeStr=boolean
  Abs : Abs
  Bus Creator : BusCreator  Inputs=6  OutDataTypeStr=Bus: vehStatesBus  NonVirtualBus=on
  Bus Selector : BusSelector  OutputSignals=InertFrm.Cg.Disp.Y,BdyFrm.Cg.Vel.ydot,InertFrm.Cg.Ang.psi,BdyFrm.Cg.AngVel.r,InertFrm.RearAxl.Disp.X,InertFrm.RearAxl.Vel.Xdot
  Compare To Constant2 : simulink/Logic and Bit Operations/Compare To Constant  relop=>=  const=4  OutDataTypeStr=boolean
  Delay : Delay
  Detect Change : simulink/Logic and Bit Operations/Detect Change  vinit=0  OutDataTypeStr=boolean
  Gain : Gain  Gain=m/2
  Lateral Control : Subsystem
  Mux1 : Mux  Inputs=6
  NOT : Logic  Operator=NOT  IconShape=distinctive  AllPortsSameDT=off  OutDataTypeStr=boolean
  OR : Logic  Operator=OR  IconShape=distinctive  AllPortsSameDT=off  OutDataTypeStr=boolean
  On Delay : powerlib_meascontrol/Logic/On Delay  DelayType=On delay  delay=1  ic=0  Ts=0
      settings: SourceProductName=Simscape Electrical
  On Delay1 : powerlib_meascontrol/Logic/On Delay  DelayType=On delay  delay=0.1  ic=0  Ts=0
      settings: SourceProductName=Simscape Electrical
  Regular Vehicle Following : Subsystem
  Subsystem : Subsystem
  Subsystem1 : Subsystem
  Subsystem2 : Subsystem
  Subsystem3 : Subsystem
  Sum1 : Sum  Inputs=|+-
  Terminator : Terminator
  Transport Delay1 : TransportDelay  DelayTime=0.01
  Triggered Subsystem : Subsystem  TreatAsAtomicUnit=on
  Vehicle Body 3DOF Single Track : autolibshared/Vehicle Body 3DOF Single Track  trackMode=Single (bicycle)  inputMode=External longitudinal forces  frontSteerMode=on  rearSteerMode=off  windMode=off  muMode=off  extFMode=off  extMMode=off  extXo=off  extpsio=off  extxdoto=off  extro=off  extYo=off  extTamb=off  extydoto=off  aMode=2  NF=2  NR=2  m=m  a=lf  b=lr  h=0.35  X_o=x0  xdot_o=vx0  CalphaMode=off  sigmaMode=on  d=0  w=[1.4,1.4]  Cy_f=12e3  Cy_r=11e3  sigma_f=.1  sigma_r=.1  alpha_f_brk=[-.1 .1]  Cy_f_data=[-9e3 9e3]  alpha_r_brk=[-.1 .1]  Cy_r_data=[-9e3 9e3]  Y_o=y0  ydot_o=0  Izz=4000  psi_o=0  r_o=0  Af=2  Cd=.3  Cl=.1  Cpm=.1  beta_w=[0:0.01:0.3]  Cs=[0:0.03:0.9]  Cym=[0:0.01:0.3]  Pabs=101325  Tair=273  g=9.81  mu=1  xdot_tol=.01  Fznom=5000  Fxtire_sat=7e4  Fytire_sat=7e4  longOff=0  latOff=0  vertOff=0  wrapAng=off
      settings: SourceProductName=Powertrain Blockset  SourceProductBaseCode=PW
  Virtual Vehicle Following : Subsystem  TreatAsAtomicUnit=on
  controlChoice : Subsystem
  findLeader : Subsystem
  followerErrors : Subsystem
  lat states : Scope  NumInputPorts=4
  maneuverState : Subsystem
  posInPlatoon : Constant  Value=posInPlatoon
  realLeader : Scope
  safeErrors : Subsystem
  strategy : Constant  Value=strategy
  system state : Scope
  vehWidth/2 : simulink/Logic and Bit Operations/Compare To Constant  relop=<=  const=0.9  OutDataTypeStr=boolean
  virtualVehiclesManager : Subsystem  TreatAsAtomicUnit=on
  states : Outport
  errors : Outport  Port=2
  virtualErrors : Outport  Port=3
  gap : Outport  Port=4
  virtualGap : Outport  Port=5
  state : Outport  Port=6
  wires:
  gapRequest/1 -> OR/2
  OR/1 -> [longAdj]
  virtualVehiclesManager/2(leaderChange) -> Virtual Vehicle Following/3(leaderChange)
  On Delay1/1 -> virtualVehiclesManager/4(lcDone)
  [longAdj] -> Virtual Vehicle Following/Enable, AND/1, virtualVehiclesManager/2(longAdj)
  controlChoice/1(u) -> Transport Delay1/1
  [state] -> controlChoice/1(state)
  vehWidth/2/1 -> NOT/1, maneuverState/5(lcDone), On Delay1/1
  safeErrors/1(safetyFlag) -> maneuverState/3(safeToVirtualFoll)
  Subsystem1/1(longAdjDone) -> maneuverState/2(steadyState)
  [longAdj] -> maneuverState/1(longAdj), maneuverState/Enable
  virtualVehiclesManager/3(virtualFollower) -> followerErrors/2(follower)
  virtualVehiclesManager/1(virtualLeader) -> Virtual Vehicle Following/2(virtualLeader)
  posInPlatoon/1 -> Subsystem2/1(posInPlatoon), virtualVehiclesManager/5(posInPlatoon)
  [state] -> Subsystem/2(state)
  NOT/1 -> Triggered Subsystem/Trigger
  On Delay/1 -> Subsystem1/4(extraSpaceFlag)
  findLeader/2(leaderIdx) -> realLeader/1, Detect Change/1
  findLeader/1(leader) -> Regular Vehicle Following/2(leader)
  Regular Vehicle Following/4(leaderInRange) -> controlChoice/3(leaderInRange)
  Subsystem/1(sat(u)) -> controlChoice/4(virtualFollControl)
  Detect Change/1 -> Regular Vehicle Following/3(leaderChange)
  Virtual Vehicle Following/2(virtualErrors) -> Subsystem1/3(virtualErrors), virtualErrors/1
  Sum1/1 -> Abs/1  "ey"
  Transport Delay1/1 -> Bus Creator/5, Subsystem1/1(u), Gain/1  "u"
  Bus Creator/1 -> states/1, followerErrors/1(ego), Virtual Vehicle Following/1(ego), findLeader/1(ego), Regular Vehicle Following/1(ego)
  latRef/1 -> Lateral Control/4(yRef), Sum1/1
  Bus Selector/4 -> Lateral Control/2(<r>), lat states/4  "<r>"
  Bus Selector/3 -> lat states/3, Bus Creator/4  "<psi>"
  Bus Selector/2 -> lat states/2  "<ydot>"
  Bus Selector/1 -> Sum1/2, Lateral Control/1(<Y>), lat states/1, Bus Creator/2  "<Y>"
  Mux1/1 -> Terminator/1
  Vehicle Body 3DOF Single Track/7 -> Mux1/6
  Vehicle Body 3DOF Single Track/6 -> Mux1/5
  Vehicle Body 3DOF Single Track/5 -> Mux1/4
  Vehicle Body 3DOF Single Track/2 -> Mux1/1
  Vehicle Body 3DOF Single Track/3 -> Mux1/2
  Vehicle Body 3DOF Single Track/4 -> Mux1/3
  Vehicle Body 3DOF Single Track/1 -> Bus Selector/1
  Gain/1 -> Vehicle Body 3DOF Single Track/3, Vehicle Body 3DOF Single Track/2
  Bus Selector/5 -> Bus Creator/1  "<X>"
  Bus Selector/6 -> Bus Creator/3  "<Xdot>"
  AND/1 -> Virtual Vehicle Following/4(extraSpaceFlag), On Delay/1, Regular Vehicle Following/4(extraSpaceFlag)  "extraSpaceFlag"
  Abs/1 -> vehWidth/2/1
  allVehicles/1 -> findLeader/2(all), virtualVehiclesManager/1(all)
  followerErrors/1(errors) -> safeErrors/1(errors)
  Regular Vehicle Following/3(gap) -> gap/1
  Regular Vehicle Following/1(u) -> controlChoice/2(follControl)
  Virtual Vehicle Following/1(u) -> Subsystem/1(u)
  Regular Vehicle Following/2(errors) -> Subsystem1/2(errors), errors/1
  Compare To Constant2/1 -> Lateral Control/3(startLaneChange)
  Lateral Control/1(delta) -> Vehicle Body 3DOF Single Track/1, Bus Creator/6
  maneuverState/1(state) -> system state/1, [state], Delay/1
  Virtual Vehicle Following/3(virtualGap) -> virtualGap/1
  [state] -> Compare To Constant2/1
  platoonState/1 -> Subsystem3/2(platoonStates), Subsystem2/3(platoonState)
  Subsystem2/1(longAdj) -> OR/1
  Delay/1 -> state/1  "u"
  strategy/1 -> Subsystem2/2(strategy), Subsystem3/1(strategy), virtualVehiclesManager/6(lcStrategy)
  Subsystem3/1(Out1) -> maneuverState/4(canStartLC)
  [state] -> findLeader/4(state)
  Virtual Vehicle Following/4(vLeaderInRange) -> controlChoice/5(vLeaderInRange)
  Triggered Subsystem/1(lcFlag) -> AND/2, findLeader/3(lcFlag), virtualVehiclesManager/3(lcFlag), Subsystem2/Enable
